simulink model "P1_T2"  (R2023a)
settings: Solver=VariableStepAuto  StartTime=0.0  StopTime=10  RelTol=1e-3
values from neighbouring files (symbols this model uses):
  Rad = Data_input(i, 2)    [script_P1_T2.m]
  Vel = Data_input(i, 1)    [script_P1_T1.m]    (also in script_P1_T2.m)
settings Model: Creator=azzam  LastModifiedBy=azzam

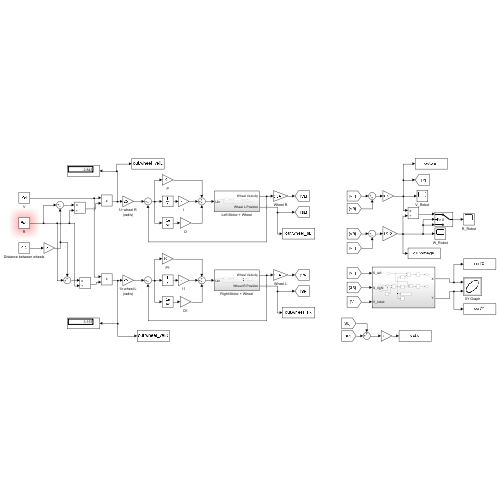
[thumbnail: Simulink's stored preview of the top-level diagram]
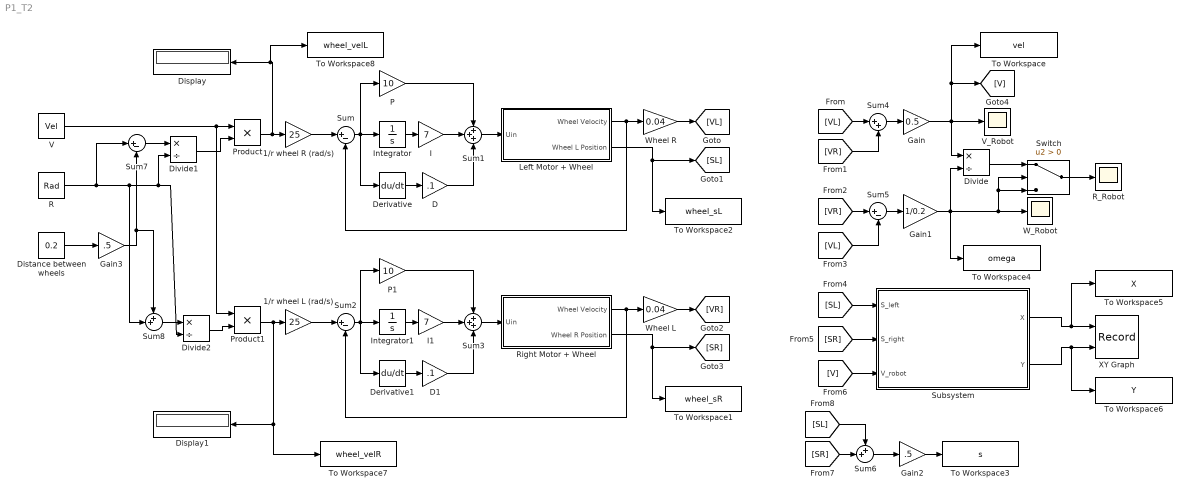
== system P1_T2 ==
  1/r wheel L (rad/s) : Gain  Gain=25
  1/r wheel R (rad/s) : Gain  Gain=25
  D : Gain  Gain=.1
  D1 : Gain  Gain=.1
  Derivative : Derivative
  Derivative1 : Derivative
  Display : Display
  Display1 : Display
  Distance between wheels : Constant  Value=0.2
  Divide : Product  Inputs=*/
  Divide1 : Product  Inputs=*/
  Divide2 : Product  Inputs=*/
  Gain : Gain  Gain=0.5
  Gain1 : Gain  Gain=1/0.2
  Gain2 : Gain  Gain=.5
  Gain3 : Gain  Gain=.5
  I : Gain  Gain=7
  I1 : Gain  Gain=7
  Integrator : Integrator
  Integrator1 : Integrator
  Left Motor + Wheel : Subsystem
  P : Gain  Gain=10
  P1 : Gain  Gain=10
  Product : Product
  Product1 : Product
  R : Constant  Value=Rad
  R_Robot : Scope
  Right Motor + Wheel : Subsystem
  Subsystem : Subsystem
  Sum{,2,5,7} (4 alike) : Sum  Inputs=|+-
  Sum1 : Sum  Inputs=+++
  Sum3 : Sum  Inputs=+++
  Sum4 : Sum  Inputs=|++
  Sum6 : Sum  Inputs=++|
  Sum8 : Sum  Inputs=++|
  Switch : Switch  Criteria=u2 > Threshold  SaturateOnIntegerOverflow=off  InputSameDT=off
  To Workspace : ToWorkspace  VariableName=vel  SaveFormat=Timeseries  SampleTime=-1
  To Workspace1 : ToWorkspace  VariableName=wheel_sR  SaveFormat=Timeseries  SampleTime=-1
  To Workspace2 : ToWorkspace  VariableName=wheel_sL  SaveFormat=Timeseries  SampleTime=-1
  To Workspace3 : ToWorkspace  VariableName=s  SaveFormat=Timeseries  SampleTime=-1
  To Workspace4 : ToWorkspace  VariableName=omega  SaveFormat=Timeseries  SampleTime=-1
  To Workspace5 : ToWorkspace  VariableName=X  SampleTime=-1
      settings: Save2DSignal=2-D array (concatenate along first dimension)
  To Workspace6 : ToWorkspace  VariableName=Y  SampleTime=-1
  To Workspace7 : ToWorkspace  VariableName=wheel_velR  SaveFormat=Timeseries  SampleTime=-1
  To Workspace8 : ToWorkspace  VariableName=wheel_velL  SaveFormat=Timeseries  SampleTime=-1
  V : Constant  Value=Vel
  V_Robot : Scope
  W_Robot : Scope
  Wheel L : Gain  Gain=0.04
  Wheel R : Gain  Gain=0.04
  XY Graph : Record  FileSettingsInternal="{\"entries\":[{\"content\":{\"excelSettings\":{\"content\":{},\"type\":\"Streamout.ExcelSettings\"}},\"type\":\"Streamout.FileSettingStorage\",\"uuid\":\"\"}],\"packageUris\":[\"http:\\/\\/schema.mathworks.com\\/mf0\\/streamout_blocks\\/R2020a\"],\"version\":\"1.0\"}"  Layout=[1 1]  SignalsInternal="{\"entries\":[{\"content\":{\"signals\":[{\"content\":{\"blockPath\":[],\"dimensions\":[1],\"domain\":\"\",\"lineColor\":\"#0072bd\",\"port\":1,\"sid\":[\"\"],\"signalID\":6510,\"signalName\":\"Subsystem:1\"},\"type\":\"RecordBlkView.Signal\",\"uuid\":\"\"},{\"content\":{\"blockPath\":[],\"dimensions\":[1],\"domain\":\"\",\"lineColor\":\"#d95319\",\"port\":2,\"sid\":[\"\"],\"signalID\":6514,\"signalName\":\"Subsystem:2\"},\"type\":\"RecordBlkView.Signal\",\"uuid\":\"\"}]},\"type\":\"RecordBlkView.InputSignals\",\"uuid\":\"\"}],\"packageUris\":[\"http:\\/\\/schema.mathworks.com\\/mf0\\/streamout_blocks\\/R2020a\"],\"version\":\"1.0\"}"  VisualizationBindings="{\"xyplotplugin\":{\"info\":[{\"series\":[],\"subplotID\":1}]}}"  CompatibilityTag=XY
  wires:
  1/r wheel R (rad/s)/1 -> Sum/1
  Integrator/1 -> I/1
  Derivative/1 -> D/1
  Sum/1 -> Derivative/1, P/1, Integrator/1
  P/1 -> Sum1/1
  I/1 -> Sum1/2
  D/1 -> Sum1/3
  Sum1/1 -> Left Motor + Wheel/1(Uin)
  Left Motor + Wheel/1(Wheel Velocity) -> Sum/2, Wheel R/1
  Wheel R/1 -> [VL]
  Left Motor + Wheel/2(Wheel L Position) -> To Workspace2/1, [SL]
  Wheel L/1 -> [VR]
  Right Motor + Wheel/1(Wheel Velocity) -> Sum2/2, Wheel L/1
  Sum3/1 -> Right Motor + Wheel/1(Uin)
  D1/1 -> Sum3/3
  P1/1 -> Sum3/1
  Derivative1/1 -> D1/1
  Sum2/1 -> Derivative1/1, P1/1, Integrator1/1
  Integrator1/1 -> I1/1
  I1/1 -> Sum3/2
  1/r wheel L (rad/s)/1 -> Sum2/1
  Right Motor + Wheel/2(Wheel R Position) -> To Workspace1/1, [SR]
  [VL] -> Sum4/1
  [VR] -> Sum4/2
  Sum4/1 -> Gain/1
  [VR] -> Sum5/1
  [VL] -> Sum5/2
  Sum5/1 -> Gain1/1
  Gain/1 -> To Workspace/1, [V], V_Robot/1, Divide/1
  Gain1/1 -> To Workspace4/1, Switch/3, Switch/2, W_Robot/1, Divide/2
  Divide/1 -> Switch/1
  Switch/1 -> R_Robot/1
  [SL] -> Subsystem/1(S_left)
  [SR] -> Subsystem/2(S_right)
  [V] -> Subsystem/3(V_robot)
  Subsystem/1(X) -> To Workspace5/1, XY Graph/1
  Subsystem/2(Y) -> To Workspace6/1, XY Graph/2
  [SR] -> Sum6/2
  [SL] -> Sum6/1
  Sum6/1 -> Gain2/1
  Gain2/1 -> To Workspace3/1
  Product/1 -> To Workspace8/1, Display/1, 1/r wheel R (rad/s)/1
  Product1/1 -> To Workspace7/1, Display1/1, 1/r wheel L (rad/s)/1
  V/1 -> Product/1, Product1/1
  Divide1/1 -> Product/2
  Sum7/1 -> Divide1/1
  R/1 -> Sum8/2, Divide1/2, Divide2/2, Sum7/1
  Distance between wheels/1 -> Gain3/1
  Gain3/1 -> Sum8/1, Sum7/2
  Sum8/1 -> Divide2/1
  Divide2/1 -> Product1/2

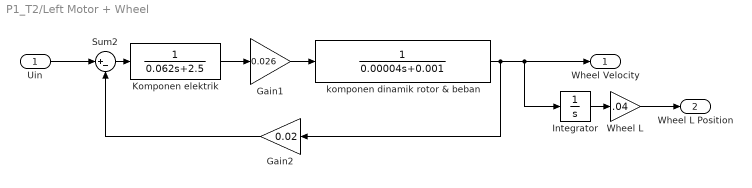
== system P1_T2/Left Motor + Wheel ==
  Uin : Inport
  Gain1 : Gain  Gain=0.026
  Gain2 : Gain  Gain=0.02
  Integrator : Integrator
  Komponen elektrik : TransferFcn  Denominator=[0.062 2.5]
  Sum2 : Sum  Inputs=|+-
  Wheel L : Gain  Gain=.04
  komponen dinamik rotor & beban : TransferFcn  Denominator=[0.00004 0.001]
  Wheel Velocity : Outport
  Wheel L Position : Outport  Port=2
  wires:
  Sum2/1 -> Komponen elektrik/1
  Komponen elektrik/1 -> Gain1/1
  Gain2/1 -> Sum2/2
  Gain1/1 -> komponen dinamik rotor & beban/1
  Uin/1 -> Sum2/1
  komponen dinamik rotor & beban/1 -> Gain2/1, Integrator/1, Wheel Velocity/1
  Integrator/1 -> Wheel L/1
  Wheel L/1 -> Wheel L Position/1

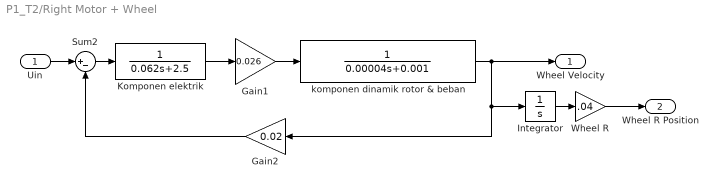
== system P1_T2/Right Motor + Wheel ==
  Uin : Inport
  Gain1 : Gain  Gain=0.026
  Gain2 : Gain  Gain=0.02
  Integrator : Integrator
  Komponen elektrik : TransferFcn  Denominator=[0.062 2.5]
  Sum2 : Sum  Inputs=|+-
  Wheel R : Gain  Gain=.04
  komponen dinamik rotor & beban : TransferFcn  Denominator=[0.00004 0.001]
  Wheel Velocity : Outport
  Wheel R Position : Outport  Port=2
  wires:
  Uin/1 -> Sum2/1
  Integrator/1 -> Wheel R/1
  Wheel R/1 -> Wheel R Position/1
  Gain1/1 -> komponen dinamik rotor & beban/1
  Komponen elektrik/1 -> Gain1/1
  Gain2/1 -> Sum2/2
  Sum2/1 -> Komponen elektrik/1
  komponen dinamik rotor & beban/1 -> Gain2/1, Integrator/1, Wheel Velocity/1

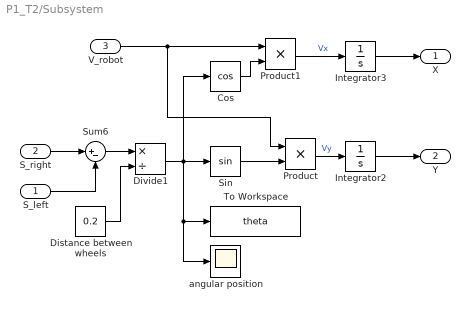
== system P1_T2/Subsystem ==
  S_left : Inport
  S_right : Inport  Port=2
  V_robot : Inport  Port=3
  Cos : Trigonometry  Operator=cos
  Distance between wheels : Constant  Value=0.2
  Divide1 : Product  Inputs=*/
  Integrator2 : Integrator
  Integrator3 : Integrator
  Product : Product
  Product1 : Product
  Sin : Trigonometry
  Sum6 : Sum  Inputs=|+-
  To Workspace : ToWorkspace  VariableName=theta  SaveFormat=Timeseries  SampleTime=-1
  angular position : Scope
  X : Outport
  Y : Outport  Port=2
  wires:
  Sin/1 -> Product/2
  V_robot/1 -> Product1/1, Product/1
  Divide1/1 -> angular position/1, To Workspace/1, Cos/1, Sin/1
  S_left/1 -> Sum6/2
  Product/1 -> Integrator2/1  "Vy"
  Integrator3/1 -> X/1
  Product1/1 -> Integrator3/1  "Vx"
  Integrator2/1 -> Y/1
  Sum6/1 -> Divide1/1
  Cos/1 -> Product1/2
  S_right/1 -> Sum6/1
  Distance between wheels/1 -> Divide1/2
